simulink model "computer_server_backplane_power"  (R2016a)
settings: Solver=ode15s  StartTime=0.0  StopTime=0.2  MaxStep=1/fs1  RelTol=1/fs
values from neighbouring files (symbols this model uses):
  C = 680e-6    (= 0.00068)    [parameters.m]
  C1 = 220e-6    (= 0.00022)    [parameters.m]
  Cf = 0.01e-6    (= 1e-08)    [parameters.m]
  D1 = 1-Vg1/Vo1    [parameters.m]
  Dmax = 0.9    [parameters.m]
  Dmin = 0    [parameters.m]
  fline = 50    [parameters.m]
  fs = 200e3    (= 200000)    [parameters.m]
  fs1 = 1e5    (= 100000)    [parameters.m]
  Gci0 = Gciwc/abs(1+wzc/(i*wc1))    [parameters.m]
  Gcv0 = Gcvwc/abs(1+wz/(i*wc))    [parameters.m]
  Gcv01 = Gcvwv/abs(1+wzo/(i*wv))    [parameters.m]
  H = 0.6    [parameters.m]
  H1 = 1/100    (= 0.01)    [parameters.m]
  Io = Pout/Vo    (= 41.6666666667)    [parameters.m]
  L = 45e-6    (= 4.5e-05)    [parameters.m]
  L1 = 250e-6    (= 0.00025)    [parameters.m]
  n = V1dc/V2dc    (= 8.33333333333)    [parameters.m]
  Pout = 500    [parameters.m]
  Resr = 0.5e-3    (= 0.0005)    [parameters.m]
  RL = 15e-3    (= 0.015)    [parameters.m]
  Rload = Vo/Io    (= 0.288)    [parameters.m]
  Rload1 = Vo1^2/Pout    (= 320)    [parameters.m]
  Rs = 0.1    [parameters.m]
  Rs1 = 0.25    [parameters.m]
  Va = Rs*ma*(1/fs)    (= 0.133333333333)    [parameters.m]
  Vac = 240    [parameters.m]
  Vcc = 12    [parameters.m]
  Vcmax = 12    [parameters.m]
  Vg1 = Vac*sqrt(2)    [parameters.m]
  VM = 1/3    (= 0.333333333333)    [parameters.m]
  Vo = 12    [parameters.m]
  Vo1 = 400    [parameters.m]
  Voffset = 0    [parameters.m]
  Vp = 3    [parameters.m]
  wz = 2*pi*fz    (= 251.327412287)    [parameters.m]
  wzc = 2*pi*fzc    (= 12566.3706144)    [parameters.m]
  wzo = 2*pi*fzo    (= 2094.39510239)    [parameters.m]
libraries: powerlib x10, simulink x5, simulink_extras x1
settings Model: Creator=Gorkem  LastModifiedBy=Gorkem
settings GRTTargetCC: GeneratePreprocessorConditionals=Use local settings

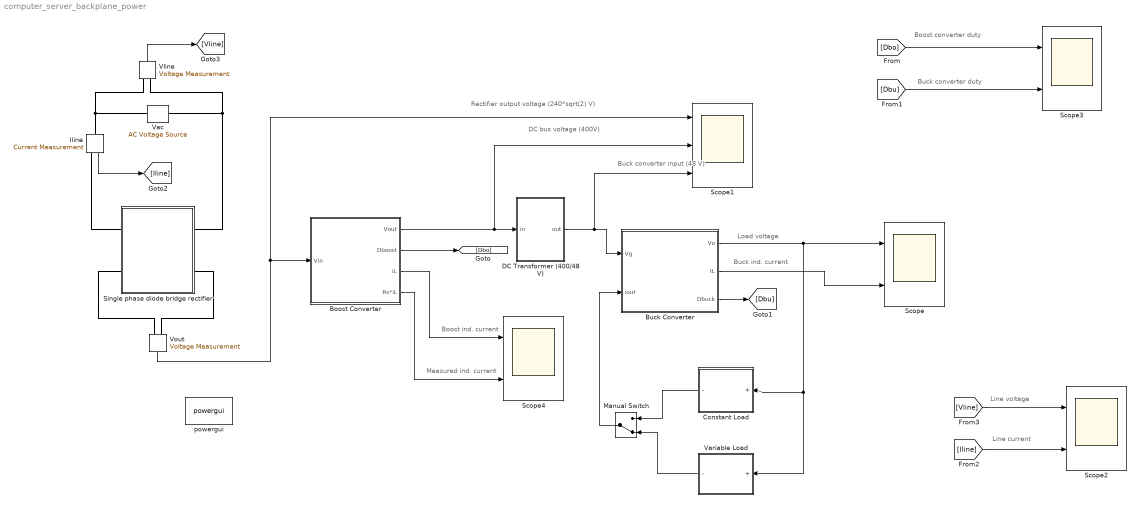
== system computer_server_backplane_power ==
  note: Buck ind. current
  note: Load voltage
  note: Measured ind. current
  note: Boost ind. current
  note: Line current
  note: Line voltage
  note: Buck converter duty
  note: Boost converter duty
  note: Buck converter input
      |
      |             (48 V)
  note: DC bus voltage (400V)
  note: Rectifier output voltage (240*sqrt(2) V)
  Boost Converter : Subsystem
  Buck Converter : Subsystem
  Constant Load : Subsystem
  DC Transformer (400/48 V) : Subsystem
  Iline : powerlib/Measurements/Current Measurement  PhasorSimulation=off  OutputType=Complex  PSBequivalent=0
  Manual Switch : ManualSwitch  CurrentSetting=0
  Scope{,2..4} (4 alike) : Scope  NumInputPorts=2
  Scope1 : Scope  NumInputPorts=3
  Single phase diode bridge rectifier : Subsystem
  Vac : powerlib/Electrical Sources/AC Voltage Source  Amplitude=Vac*sqrt(2)  Phase=0  Frequency=fline  SampleTime=0  Measurements=Voltage  BusType=swing  Pref=10e3  Qref=0  Qmin=-inf  Qmax=+inf
  Variable Load : Subsystem
  Vline : powerlib/Measurements/Voltage Measurement  PhasorSimulation=off  OutputType=Complex  PSBequivalent=0
  Vout : powerlib/Measurements/Voltage Measurement  PhasorSimulation=off  OutputType=Complex  PSBequivalent=0
  powergui : powerlib/powergui  Priority=1  SimulationMode=Continuous  SolverType=Tustin/Backward Euler (TBE)  SampleTime=50e-6  frequency=50  SPID=on  DisableSnubberDevices=on  DisableRonSwitches=off  DisableVfSwitches=off  SwTol=0  DisplayEquations=off  Interpol=off  ExternalGateDelay=off  methode=off  Ts=10  FunctionMessages=off  echomessages=off  HookPort=off  EnableUseOfTLC=off  x0status=blocks  frequencyindice=50  Pbase=100e6  ErrMax=1e-4  Iterations=50  UnitsV=kV  UnitsW=MW  buscounter=0  RestoreLinks=warning  ResistiveCurrentMeasurement=off  Frange=[0:2:500]  Ylog=off  Xlog=on  ShowGrid=off  save=off  variable=ZData  structure=0  ZoomFFT=off  StartTime=0.0  cycles=1  DisplayStyle=1  fundamental=60  FreqAxis=off  MaxFrequency=1000  frequencyindicesteady=1  RmsSteady=1  display=off
  wires:
  Buck Converter/1(Vo) -> Constant Load/1(+), Variable Load/1(+), Scope/1
  Buck Converter/2(IL) -> Scope/2
  DC Transformer (400/48 V)/1(out) -> Buck Converter/1(Vg), Scope1/3
  Boost Converter/1(Vout) -> DC Transformer (400/48 V)/1(in), Scope1/2
  Vout/1 -> Scope1/1, Boost Converter/1(Vin)
  Constant Load/1(-) -> Manual Switch/1
  Variable Load/1(-) -> Manual Switch/2
  Manual Switch/1 -> Buck Converter/2(iout)
  Boost Converter/2(Dboost) -> [Dbo]
  [Dbo] -> Scope3/1
  Buck Converter/3(Dbuck) -> [Dbu]
  [Dbu] -> Scope3/2
  Iline/1 -> [Iline]
  Vline/1 -> [Vline]
  [Vline] -> Scope2/1
  [Iline] -> Scope2/2
  Boost Converter/3(iL) -> Scope4/1
  Boost Converter/4(Rs*iL) -> Scope4/2
  connections:
  Vout/LConn1 -- Single phase diode bridge rectifier/LConn2
  Vout/LConn2 -- Single phase diode bridge rectifier/RConn2
  Vac/LConn1 -- Single phase diode bridge rectifier/RConn1 -- Vline/LConn2
  Iline/LConn1 -- Vline/LConn1 -- Vac/RConn1
  Iline/RConn1 -- Single phase diode bridge rectifier/LConn1

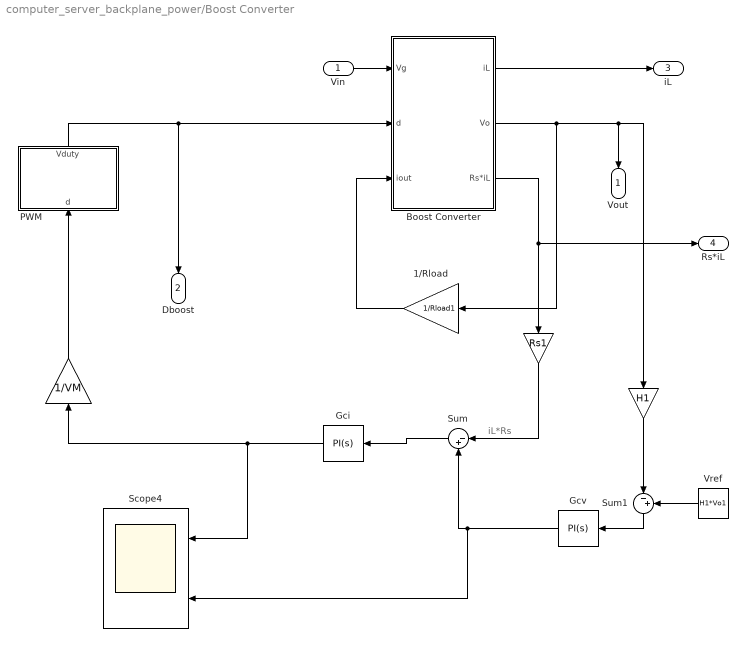
== system computer_server_backplane_power/Boost Converter ==
  note: iL*Rs
  Vin : Inport
  "  " : Gain  Gain=Rs1
  "     " : Gain  Gain=1/VM
  "           " : Gain  Gain=H1
  "  1/Rload" : Gain  Gain=1/Rload1
  Boost Converter : Subsystem
  Gci : simulink/Continuous/PID Controller  Controller=PI  TimeDomain=Continuous-time  SampleTime=-1  IntegratorMethod=Forward Euler  FilterMethod=Forward Euler  Form=Parallel  UseFilter=on  ControllerParametersSource=internal  P=Gci0  I=Gci0*wzc  D=0  N=100  InitialConditionSource=internal  InitialConditionForIntegrator=0  InitialConditionForFilter=0  ExternalReset=none  LimitOutput=on  UpperSaturationLimit=D1  LowerSaturationLimit=0.25*D1  LinearizeAsGain=off  AntiWindupMode=none  Kb=1  TrackingMode=off  Kt=1  PParamMin=[]  PParamMax=[]  IParamMin=[]  IParamMax=[]  DParamMin=[]  DParamMax=[]  NParamMin=[]  NParamMax=[]  KbParamMin=[]  KbParamMax=[]  KtParamMin=[]  KtParamMax=[]  POutMin=[]  POutMax=[]  IOutMin=[]  IOutMax=[]  DOutMin=[]  DOutMax=[]  NOutMin=[]  NOutMax=[]  KbOutMin=[]  KbOutMax=[]  KtOutMin=[]  KtOutMax=[]  IntegratorOutMin=[]  IntegratorOutMax=[]  FilterOutMin=[]  FilterOutMax=[]  SumOutMin=[]  SumOutMax=[]  SumI1OutMin=[]  SumI1OutMax=[]  SumI2OutMin=[]  SumI2OutMax=[]  SumI3OutMin=[]  SumI3OutMax=[]  SumDOutMin=[]  SumDOutMax=[]  SaturationOutMin=[]  SaturationOutMax=[]  IntegratorContinuousStateAttributes=''  IntegratorStateMustResolveToSignalObject=off  IntegratorRTWStateStorageClass=Auto  FilterContinuousStateAttributes=''  FilterStateMustResolveToSignalObject=off  FilterRTWStateStorageClass=Auto  DifferentiatorICPrevScaledInput=0  DifferentiatorOutMin=[]  DifferentiatorOutMax=[]
  Gcv : simulink/Continuous/PID Controller  Controller=PI  TimeDomain=Continuous-time  SampleTime=-1  IntegratorMethod=Forward Euler  FilterMethod=Forward Euler  Form=Parallel  UseFilter=on  ControllerParametersSource=internal  P=Gcv01  I=Gcv01*wzo  D=0  N=100  InitialConditionSource=internal  InitialConditionForIntegrator=0  InitialConditionForFilter=0  ExternalReset=none  LimitOutput=on  UpperSaturationLimit=Rs1*(Pout/Vg1)  LowerSaturationLimit=0.8*Rs1*(Pout/Vg1)  LinearizeAsGain=off  AntiWindupMode=none  Kb=1  TrackingMode=off  Kt=1  PParamMin=[]  PParamMax=[]  IParamMin=[]  IParamMax=[]  DParamMin=[]  DParamMax=[]  NParamMin=[]  NParamMax=[]  KbParamMin=[]  KbParamMax=[]  KtParamMin=[]  KtParamMax=[]  POutMin=[]  POutMax=[]  IOutMin=[]  IOutMax=[]  DOutMin=[]  DOutMax=[]  NOutMin=[]  NOutMax=[]  KbOutMin=[]  KbOutMax=[]  KtOutMin=[]  KtOutMax=[]  IntegratorOutMin=[]  IntegratorOutMax=[]  FilterOutMin=[]  FilterOutMax=[]  SumOutMin=[]  SumOutMax=[]  SumI1OutMin=[]  SumI1OutMax=[]  SumI2OutMin=[]  SumI2OutMax=[]  SumI3OutMin=[]  SumI3OutMax=[]  SumDOutMin=[]  SumDOutMax=[]  SaturationOutMin=[]  SaturationOutMax=[]  IntegratorContinuousStateAttributes=''  IntegratorStateMustResolveToSignalObject=off  IntegratorRTWStateStorageClass=Auto  FilterContinuousStateAttributes=''  FilterStateMustResolveToSignalObject=off  FilterRTWStateStorageClass=Auto  DifferentiatorICPrevScaledInput=0  DifferentiatorOutMin=[]  DifferentiatorOutMax=[]
  "PWM " : Subsystem
  Scope4 : Scope  NumInputPorts=2
  Sum : Sum  Inputs=|-+
  Sum1 : Sum  Inputs=|-+
  Vref : Constant  Value=H1*Vo1
  Vout : Outport
  Dboost : Outport  Port=2
  iL : Outport  Port=3
  Rs*iL : Outport  Port=4
  wires:
  Boost Converter/1(iL) -> iL/1
  Gcv/1 -> Scope4/2, Sum/2
  Vin/1 -> Boost Converter/1(Vg)
  "  "/1 -> Sum/1
  "     "/1 -> "PWM "/1(d)
  Sum1/1 -> Gcv/1
  Sum/1 -> Gci/1
  Boost Converter/3(Rs*iL) -> Rs*iL/1, "  "/1
  "           "/1 -> Sum1/1
  Vref/1 -> Sum1/2
  Gci/1 -> Scope4/1, "     "/1
  Boost Converter/2(Vo) -> "  1/Rload"/1, Vout/1, "           "/1
  "  1/Rload"/1 -> Boost Converter/3(iout)
  "PWM "/1(Vduty) -> Dboost/1, Boost Converter/2(d)

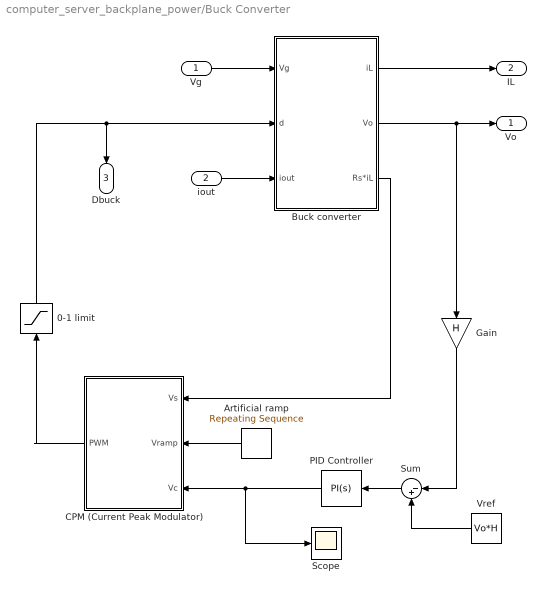
== system computer_server_backplane_power/Buck Converter ==
  Vg : Inport
  iout : Inport  Port=2
  0-1 limit : Saturate  UpperLimit=1  LowerLimit=0
  Artificial ramp : simulink/Sources/Repeating Sequence  rep_seq_t=[0 0.999/fs 1/fs]  rep_seq_y=[0 Va 0]
  Buck converter : Subsystem
  CPM (Current Peak Modulator) : Subsystem
  Gain : Gain  Gain=H
  PID Controller : simulink/Continuous/PID Controller  Controller=PI  TimeDomain=Continuous-time  SampleTime=-1  IntegratorMethod=Forward Euler  FilterMethod=Forward Euler  Form=Parallel  UseFilter=on  ControllerParametersSource=internal  P=Gcv0  I=Gcv0*wz  D=0  N=100  InitialConditionSource=internal  InitialConditionForIntegrator=0  InitialConditionForFilter=0  ExternalReset=none  LimitOutput=on  UpperSaturationLimit=Vcmax+Voffset  LowerSaturationLimit=0.8*Io*Rs  LinearizeAsGain=on  AntiWindupMode=none  Kb=1  TrackingMode=off  Kt=1  PParamMin=[]  PParamMax=[]  IParamMin=[]  IParamMax=[]  DParamMin=[]  DParamMax=[]  NParamMin=[]  NParamMax=[]  KbParamMin=[]  KbParamMax=[]  KtParamMin=[]  KtParamMax=[]  POutMin=[]  POutMax=[]  IOutMin=[]  IOutMax=[]  DOutMin=[]  DOutMax=[]  NOutMin=[]  NOutMax=[]  KbOutMin=[]  KbOutMax=[]  KtOutMin=[]  KtOutMax=[]  IntegratorOutMin=[]  IntegratorOutMax=[]  FilterOutMin=[]  FilterOutMax=[]  SumOutMin=[]  SumOutMax=[]  SumI1OutMin=[]  SumI1OutMax=[]  SumI2OutMin=[]  SumI2OutMax=[]  SumI3OutMin=[]  SumI3OutMax=[]  SumDOutMin=[]  SumDOutMax=[]  SaturationOutMin=[]  SaturationOutMax=[]  IntegratorContinuousStateAttributes=''  IntegratorStateMustResolveToSignalObject=off  IntegratorRTWStateStorageClass=Auto  FilterContinuousStateAttributes=''  FilterStateMustResolveToSignalObject=off  FilterRTWStateStorageClass=Auto  DifferentiatorICPrevScaledInput=0  DifferentiatorOutMin=[]  DifferentiatorOutMax=[]
  Scope : Scope
  Sum : Sum  Inputs=|-+
  Vref : Constant  Value=Vo*H
  Vo : Outport
  IL : Outport  Port=2
  Dbuck : Outport  Port=3
  wires:
  Artificial ramp/1 -> CPM (Current Peak Modulator)/2(Vramp)
  Buck converter/3(Rs*iL) -> CPM (Current Peak Modulator)/1(Vs)
  PID Controller/1 -> Scope/1, CPM (Current Peak Modulator)/3(Vc)
  iout/1 -> Buck converter/3(iout)
  Vref/1 -> Sum/2
  CPM (Current Peak Modulator)/1(PWM) -> 0-1 limit/1
  Gain/1 -> Sum/1
  Vg/1 -> Buck converter/1(Vg)
  Buck converter/1(iL) -> IL/1
  Sum/1 -> PID Controller/1
  Buck converter/2(Vo) -> Vo/1, Gain/1
  0-1 limit/1 -> Buck converter/2(d), Dbuck/1

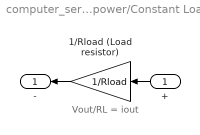
== system computer_server_backplane_power/Constant Load ==
  note: Vout/RL = iout
  + : Inport
  1/Rload (Load resistor) : Gain  Gain=1/Rload
  - : Outport
  wires:
  1/Rload (Load resistor)/1 -> -/1
  +/1 -> 1/Rload (Load resistor)/1

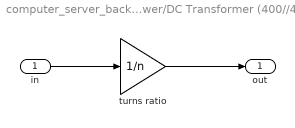
== system computer_server_backplane_power/DC Transformer (400//48 V) ==
  in : Inport
  turns ratio : Gain  Gain=1/n
  out : Outport
  wires:
  in/1 -> turns ratio/1
  turns ratio/1 -> out/1

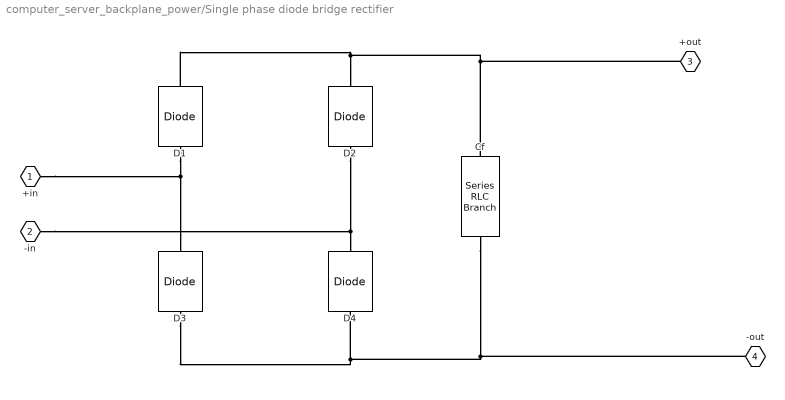
== system computer_server_backplane_power/Single phase diode bridge rectifier ==
  Cf : powerlib/Elements/Series RLC Branch  LConnTagsString=__new0  RConnTagsString=__new0  BranchType=C  Resistance=1  Inductance=1e-3  SetiL0=off  InitialCurrent=0  Capacitance=Cf  Setx0=off  InitialVoltage=0  Measurements=Branch voltage and current
  D{1..4} (4 alike) : powerlib/Power Electronics/Diode  Ron=Ron  Lon=0  Vf=Vf  IC=0  UseSnubber=off  Rs=10e6  Cs=0  Measurements=off
  +in : PMIOPort  Port=1  Side=Left
  -in : PMIOPort  Port=2  Side=Right
  +out : PMIOPort  Port=3  Side=Left
  -out : PMIOPort  Port=4  Side=Right
  connections:
  D1/LConn1 -- +in/RConn1 -- D3/RConn1
  D1/RConn1 -- +out/RConn1 -- Cf/LConn1 -- D2/RConn1
  D3/LConn1 -- Cf/RConn1 -- -out/RConn1 -- D4/LConn1
  D2/LConn1 -- -in/RConn1 -- D4/RConn1

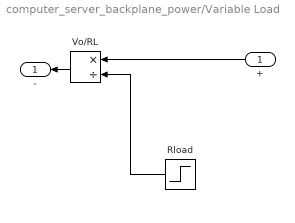
== system computer_server_backplane_power/Variable Load ==
  + : Inport
  Rload : Step  Time=0.1  Before=Rload  After=Rload/2  SampleTime=0
  Vo/RL : Product  Inputs=*/
  - : Outport
  wires:
  Vo/RL/1 -> -/1
  +/1 -> Vo/RL/1
  Rload/1 -> Vo/RL/2

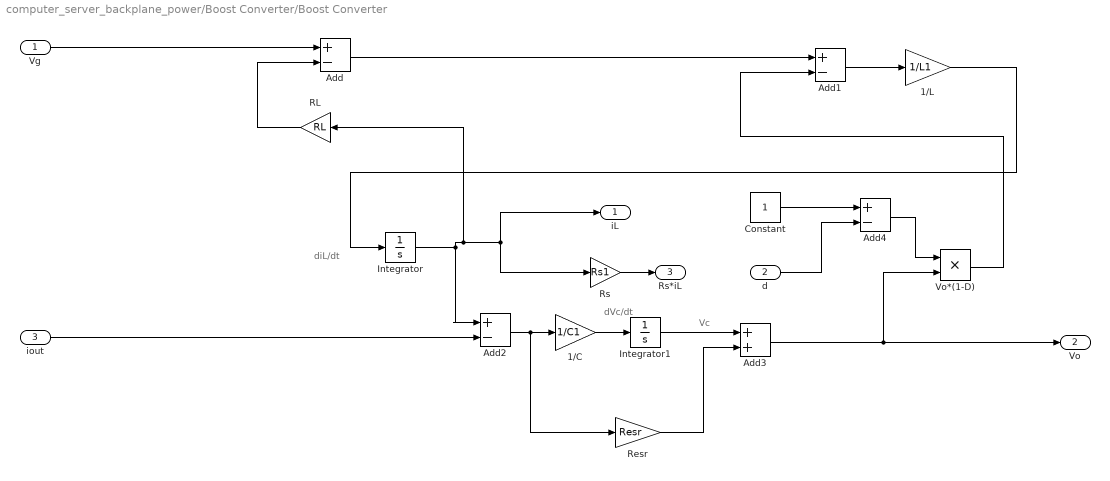
== system computer_server_backplane_power/Boost Converter/Boost Converter ==
  note: Vc
  note: dVc/dt
  note: diL/dt
  Vg : Inport
  d : Inport  Port=2
  iout : Inport  Port=3
  1/C : Gain  Gain=1/C1
  1/L : Gain  Gain=1/L1
  Add{,1..2,4} (4 alike) : Sum  Inputs=+-
  Add3 : Sum
  Constant : Constant
  Integrator : Integrator
  Integrator1 : Integrator  UpperSaturationLimit=Vo
  RL : Gain  Gain=RL
  Resr : Gain  Gain=Resr
  Rs : Gain  Gain=Rs1
  Vo*(1-D) : Product
  iL : Outport
  Vo : Outport  Port=2
  Rs*iL : Outport  Port=3
  wires:
  1/C/1 -> Integrator1/1
  Add2/1 -> Resr/1, 1/C/1
  Vg/1 -> Add/1
  Add1/1 -> 1/L/1
  Add3/1 -> Vo*(1-D)/2, Vo/1
  Integrator1/1 -> Add3/1
  Resr/1 -> Add3/2
  RL/1 -> Add/2
  iout/1 -> Add2/2
  Add/1 -> Add1/1
  Rs/1 -> Rs*iL/1
  d/1 -> Add4/2
  Integrator/1 -> Add2/1, RL/1, Rs/1, iL/1
  1/L/1 -> Integrator/1
  Constant/1 -> Add4/1
  Add4/1 -> Vo*(1-D)/1
  Vo*(1-D)/1 -> Add1/2

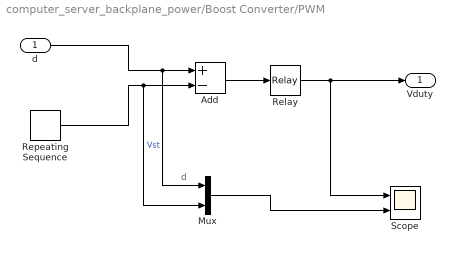
== system computer_server_backplane_power/Boost Converter/PWM  ==
  note: d
  d : Inport
  Add : Sum  Inputs=+-
  Mux : Mux  Inputs=2
  Relay : Relay  ZeroCross=off
  Repeating Sequence : simulink/Sources/Repeating Sequence  rep_seq_t=[0 0.001e-5 1/fs1]  rep_seq_y=[Vp 0 Vp]
  Scope : Scope  NumInputPorts=2
  Vduty : Outport
  wires:
  Relay/1 -> Vduty/1, Scope/1
  Repeating Sequence/1 -> Mux/2, Add/2  "Vst"
  Add/1 -> Relay/1
  Mux/1 -> Scope/2
  d/1 -> Mux/1, Add/1

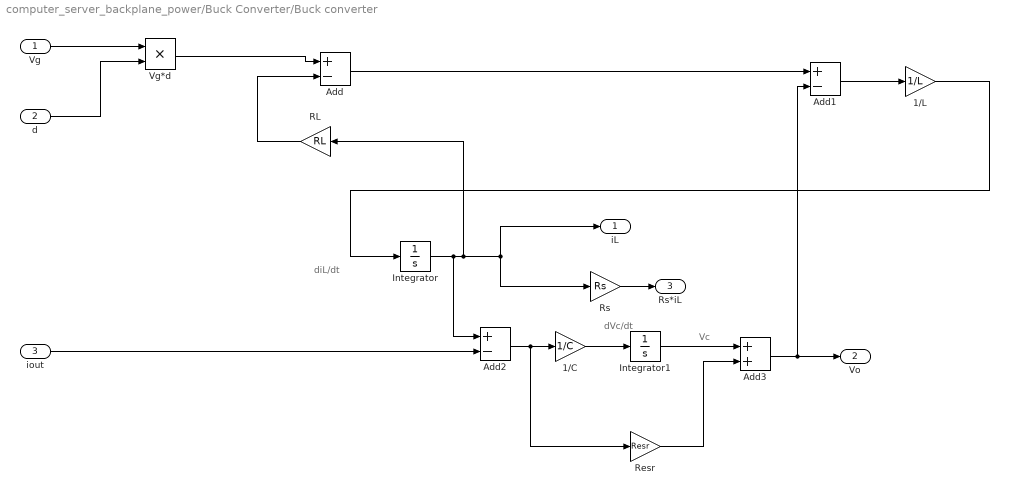
== system computer_server_backplane_power/Buck Converter/Buck converter ==
  note: Vc
  note: dVc/dt
  note: diL/dt
  Vg : Inport
  d : Inport  Port=2
  iout : Inport  Port=3
  1/C : Gain  Gain=1/C
  1/L : Gain  Gain=1/L
  Add : Sum  Inputs=+-
  Add1 : Sum  Inputs=+-
  Add2 : Sum  Inputs=+-
  Add3 : Sum
  Integrator : Integrator
  Integrator1 : Integrator
  RL : Gain  Gain=RL
  Resr : Gain  Gain=Resr
  Rs : Gain  Gain=Rs
  Vg*d : Product
  iL : Outport
  Vo : Outport  Port=2
  Rs*iL : Outport  Port=3
  wires:
  1/L/1 -> Integrator/1
  Integrator/1 -> Add2/1, Rs/1, iL/1, RL/1
  Vg/1 -> Vg*d/1
  1/C/1 -> Integrator1/1
  Add2/1 -> Resr/1, 1/C/1
  Vg*d/1 -> Add/1
  Add1/1 -> 1/L/1
  Add3/1 -> Vo/1, Add1/2
  d/1 -> Vg*d/2
  Integrator1/1 -> Add3/1
  Resr/1 -> Add3/2
  RL/1 -> Add/2
  iout/1 -> Add2/2
  Add/1 -> Add1/1
  Rs/1 -> Rs*iL/1

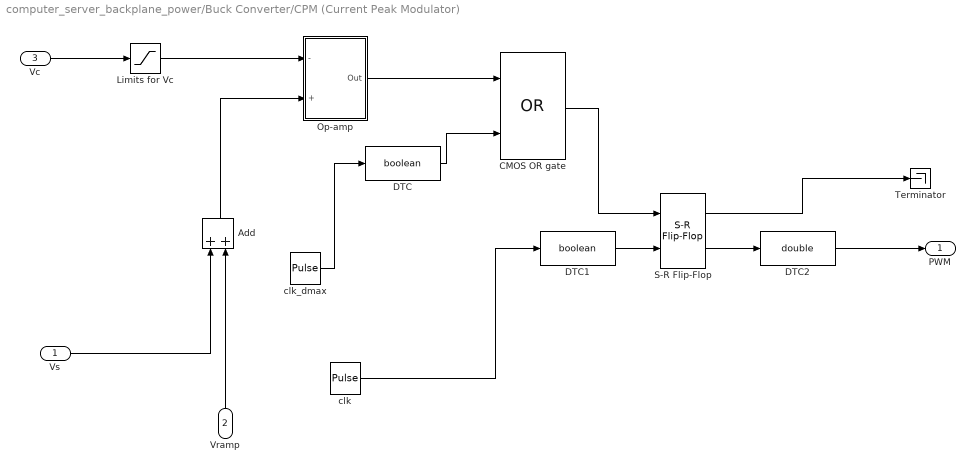
== system computer_server_backplane_power/Buck Converter/CPM (Current Peak Modulator) ==
  Vs : Inport
  Vramp : Inport  Port=2
  Vc : Inport  Port=3
  Add : Sum
  CMOS OR gate : Logic  Operator=OR  AllPortsSameDT=off  OutDataTypeStr=boolean
  DTC : DataTypeConversion  OutDataTypeStr=boolean  SaturateOnIntegerOverflow=on  LockScale=on
  DTC1 : DataTypeConversion  OutDataTypeStr=boolean  SaturateOnIntegerOverflow=on  LockScale=on
  DTC2 : DataTypeConversion  OutDataTypeStr=double  SaturateOnIntegerOverflow=on  LockScale=on
  Limits for Vc : Saturate  UpperLimit=Vcmax+Voffset  LowerLimit=0  ZeroCross=off
  Op-amp : Subsystem
  S-R Flip-Flop : simulink_extras/Flip Flops/S-R Flip-Flop  initial_condition=0
  Terminator : Terminator
  clk : DiscretePulseGenerator  PulseType=Time based  Amplitude=5  Period=1/fs  PulseWidth=(Dmin+1e-10)*100
  clk_dmax : DiscretePulseGenerator  PulseType=Time based  Amplitude=5  Period=1/fs  PulseWidth=(1-Dmax)*100  PhaseDelay=Dmax/fs
  PWM : Outport
  wires:
  Vs/1 -> Add/1
  Add/1 -> Op-amp/2(+)
  Limits for Vc/1 -> Op-amp/1(-)
  Vramp/1 -> Add/2
  Vc/1 -> Limits for Vc/1
  S-R Flip-Flop/2 -> DTC2/1
  CMOS OR gate/1 -> S-R Flip-Flop/1
  clk_dmax/1 -> DTC/1
  DTC/1 -> CMOS OR gate/2
  DTC1/1 -> S-R Flip-Flop/2
  clk/1 -> DTC1/1
  S-R Flip-Flop/1 -> Terminator/1
  Op-amp/1(Out) -> CMOS OR gate/1
  DTC2/1 -> PWM/1

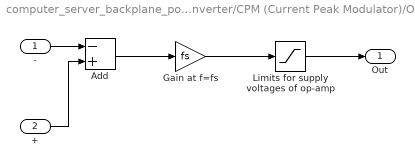
== system computer_server_backplane_power/Buck Converter/CPM (Current Peak Modulator)/Op-amp ==
  - : Inport
  + : Inport  Port=2
  Add : Sum  Inputs=-+
  Gain at f=fs : Gain  Gain=fs
  "Limits for supply voltages of op-amp " : Saturate  UpperLimit=Vcc  LowerLimit=0
  Out : Outport
  wires:
  Add/1 -> Gain at f=fs/1
  Gain at f=fs/1 -> "Limits for supply voltages of op-amp "/1
  "Limits for supply voltages of op-amp "/1 -> Out/1
  -/1 -> Add/1
  +/1 -> Add/2
